simulink model "MSICA_Projet1_StructureModaleControle"  (R2018a)
settings: Solver=VariableStepAuto  StartTime=0.0  StopTime=10.0  RelTol=1e-3
values from neighbouring files (symbols this model uses):
  A_S1_S2 = [ zeros(3,3) eye(3) ... (first row only)    [DonneesProjet.m]
  Amod = [zeros(3) eye(3); -omega_carre -2*xi*sqrt(omega_carre)]    [DonneesProjet.m]
  B_S1_S2 = [zeros(3,3); inv(M_S1_S2)]    [DonneesProjet.m]
  Bmod = [zeros(3); phi']    [DonneesProjet.m]
  C1 = [eye(3) zeros(3,3)]    [DonneesProjet.m]
  Cmod = [phi zeros(3,3)]    [DonneesProjet.m]
libraries: Blocs_LTI x2
settings Model: Creator=natha  LastModifiedBy=natha
settings DataIOCC: ReturnWorkspaceOutputs=on
settings SFSimCC: SimUseLocalCustomCode=on
settings RTWCC: RTWUseLocalCustomCode=on

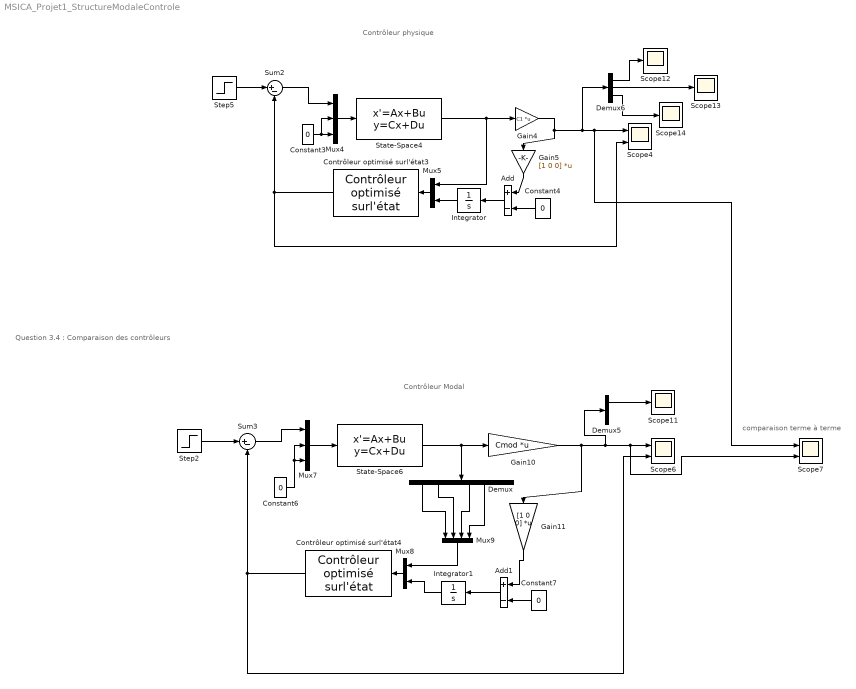
== system MSICA_Projet1_StructureModaleControle ==
  note: Contrôleur physique
  note: Contrôleur Modal
  note: Question 3.4 : Comparaison des contrôleurs
  note: comparaison terme à terme
  Add : Sum  Inputs=+-
  Add1 : Sum  Inputs=+-
  Constant{3..4,6..7} (4 alike) : Constant  Value=0
  Contrôleur optimisé surl'état3 : Blocs_LTI/Contrôleur optimisé surl'état  MaskParameter1=A2  MaskParameter2=B2  MaskParameter3=diag([1e7 1e7 1e7 1e5 1e5 1e5 1e11])  MaskParameter4=eye(1,1)
  Contrôleur optimisé surl'état4 : Blocs_LTI/Contrôleur optimisé surl'état  MaskParameter1=Amod2cont  MaskParameter2=Bcont  MaskParameter3=diag([1e7 1e7 1e5 1e5 1e11])  MaskParameter4=eye(1,1)
  Demux : Demux  Outputs=6
  Demux5 : Demux  Outputs=3
  Demux6 : Demux  Outputs=3
  Gain10 : Gain  Gain=Cmod  Multiplication=Matrix(K*u)
  Gain11 : Gain  Gain=[1 0 0]  Multiplication=Matrix(K*u)
  Gain4 : Gain  Gain=C1  Multiplication=Matrix(K*u)
  Gain5 : Gain  Gain=[1 0 0]  Multiplication=Matrix(K*u)
  Integrator : Integrator
  Integrator1 : Integrator
  Mux4 : Mux  Inputs=3
  Mux5 : Mux  Inputs=2
  Mux7 : Mux  Inputs=3
  Mux8 : Mux  Inputs=2
  Mux9 : Mux
  Scope{11..14} (4 alike) : Scope
  Scope4 : Scope  NumInputPorts=2
  Scope6 : Scope  NumInputPorts=2
  Scope7 : Scope  NumInputPorts=2
  State-Space4 : StateSpace  A=A_S1_S2  B=B_S1_S2  C=eye(6)  D=zeros(6,3)  InitialCondition=0
  State-Space6 : StateSpace  A=Amod  B=Bmod  C=eye(6)  D=zeros(6,3)  InitialCondition=0
  Step2 : Step  Time=0  After=10  SampleTime=0
  Step5 : Step  Time=0  After=10  SampleTime=0
  Sum2 : Sum  Inputs=|+-
  Sum3 : Sum  Inputs=|+-
  wires:
  Contrôleur optimisé surl'état4/1 -> Sum3/2, Scope6/2
  State-Space6/1 -> Demux/1, Gain10/1
  Demux/2 -> Mux9/2
  Add1/1 -> Integrator1/1
  Sum3/1 -> Mux7/1
  Step2/1 -> Sum3/1
  Demux/1 -> Mux9/1
  Integrator1/1 -> Mux8/2
  Constant7/1 -> Add1/2
  Constant6/1 -> Mux7/2, Mux7/3
  Gain10/1 -> Gain11/1, Demux5/1, Scope7/2, Scope6/1
  Mux8/1 -> Contrôleur optimisé surl'état4/1
  Gain11/1 -> Add1/1
  Mux7/1 -> State-Space6/1
  Demux/4 -> Mux9/3
  Demux/5 -> Mux9/4
  Mux9/1 -> Mux8/1
  Demux5/1 -> Scope11/1
  Constant3/1 -> Mux4/2, Mux4/3
  Mux4/1 -> State-Space4/1
  Step5/1 -> Sum2/1
  Gain5/1 -> Add/1
  Add/1 -> Integrator/1
  Constant4/1 -> Add/2
  Gain4/1 -> Demux6/1, Scope7/1, Scope4/1, Gain5/1
  State-Space4/1 -> Mux5/1, Gain4/1
  Demux6/1 -> Scope12/1
  Demux6/3 -> Scope14/1
  Mux5/1 -> Contrôleur optimisé surl'état3/1
  Demux6/2 -> Scope13/1
  Sum2/1 -> Mux4/1
  Integrator/1 -> Mux5/2
  Contrôleur optimisé surl'état3/1 -> Sum2/2, Scope4/2
